simulink library "Flow_Mixer"  (Simulink 8.2)
settings: Solver=ode45  StartTime=0.0  StopTime=10.0  RelTol=1e-3
libraries: simulink x2, carnot x1, simulink_extras x1
settings Model: Creator=lena.frank  LastModifiedBy=drhf

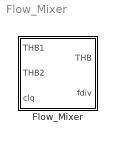
== system Flow_Mixer ==
  Flow_Mixer : Subsystem  mask(flow mixer){t=10}
      mask prompts: t "time constant of mixer"
      mask help: Mixes two massflows. The new temperature is calculated by an energy balance. The output f_div may be fed back to the corresponding flow diverter upwards in flowdirection.
      mask init:
      | if t < 0.0001
      |     t = 0.0001;
      |     disp('warning in Flow Mixer: Time constant set to 0.0001')
      | end
      mask Help: web(fullfile(path_carnot('help'),'Flow_Mixer.html'),'-helpbrowser')
      mask Display: plot(-25,-5,95,65,[20 45 20 20],[20 30 40 20],[45 70 70 45],[30 20 40 30],[45 35 55 45],[30 10 10 30])

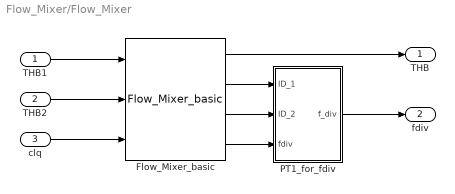
== system Flow_Mixer/Flow_Mixer ==
  THB1 : Inport
  THB2 : Inport  Port=2
  clq : Inport  Port=3
  Flow_Mixer_basic : carnot/Basic/Hydraulics/Flow_Mixer_basic
  PT1_for_fdiv : Subsystem
  THB : Outport
  fdiv : Outport  Port=2
  wires:
  clq/1 -> Flow_Mixer_basic/3
  PT1_for_fdiv/1(f_div) -> fdiv/1
  THB1/1 -> Flow_Mixer_basic/1
  THB2/1 -> Flow_Mixer_basic/2
  Flow_Mixer_basic/1 -> THB/1
  Flow_Mixer_basic/2 -> PT1_for_fdiv/1(ID_1)
  Flow_Mixer_basic/3 -> PT1_for_fdiv/2(ID_2)
  Flow_Mixer_basic/4 -> PT1_for_fdiv/3(fdiv)

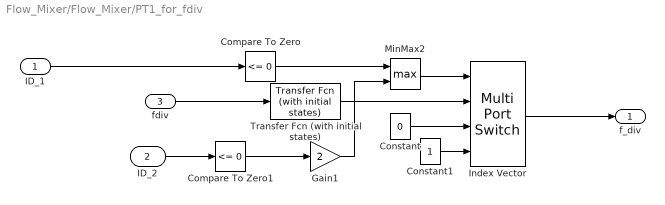
== system Flow_Mixer/Flow_Mixer/PT1_for_fdiv ==
  ID_1 : Inport
  ID_2 : Inport  Port=2
  fdiv : Inport  Port=3
  Compare To Zero : simulink/Logic and Bit Operations/Compare To Zero  relop=<=  OutDataTypeStr=uint8
  Compare To Zero1 : simulink/Logic and Bit Operations/Compare To Zero  relop=<=  OutDataTypeStr=uint8
  Constant : Constant  Value=0
  Constant1 : Constant
  Gain1 : Gain  Gain=2
  Index Vector : MultiPortSwitch  DataPortOrder=Zero-based contiguous  zeroidx=on
  MinMax2 : MinMax  Function=max  Inputs=2
  Transfer Fcn (with initial states) : simulink_extras/Additional Linear/Transfer Fcn (with initial states)  N=[1]  D="[t  1]"  X0=0.5
  f_div : Outport
  wires:
  fdiv/1 -> Transfer Fcn (with initial states)/1
  Compare To Zero1/1 -> Gain1/1
  Compare To Zero/1 -> MinMax2/1
  MinMax2/1 -> Index Vector/1
  ID_1/1 -> Compare To Zero/1
  ID_2/1 -> Compare To Zero1/1
  Constant/1 -> Index Vector/3
  Transfer Fcn (with initial states)/1 -> Index Vector/2
  Constant1/1 -> Index Vector/4
  Gain1/1 -> MinMax2/2
  Index Vector/1 -> f_div/1
